simulink model "Wheel_NoneLinear_Verif"  (R2021b)
settings: Solver=VariableStepAuto  StartTime=0.0  StopTime=10  RelTol=1e-3
values from neighbouring files (symbols this model uses):
  Kt = 14e4    (= 140000)    [CarQuarterParam.m]
  M2 = 20    [CarQuarterParam.m]
settings Model: Creator=Reece Bell  LastModifiedBy=reece
settings SolverCC: AlgebraicLoopSolver=TrustRegion
settings DataIOCC: ReturnWorkspaceOutputs=off
settings DebuggingCC: SFMachineParentedDataDiag=warning  ArithmeticOperatorsInVariantConditions=warning
settings SFSimCC: CustomCodeUndefinedFunction=UseInterfaceOnly

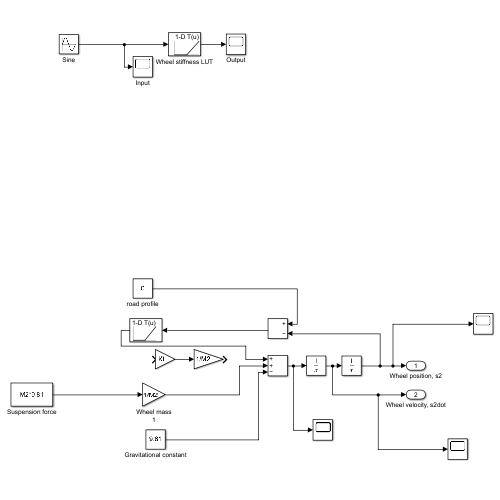
[thumbnail: Simulink's stored preview of the top-level diagram]
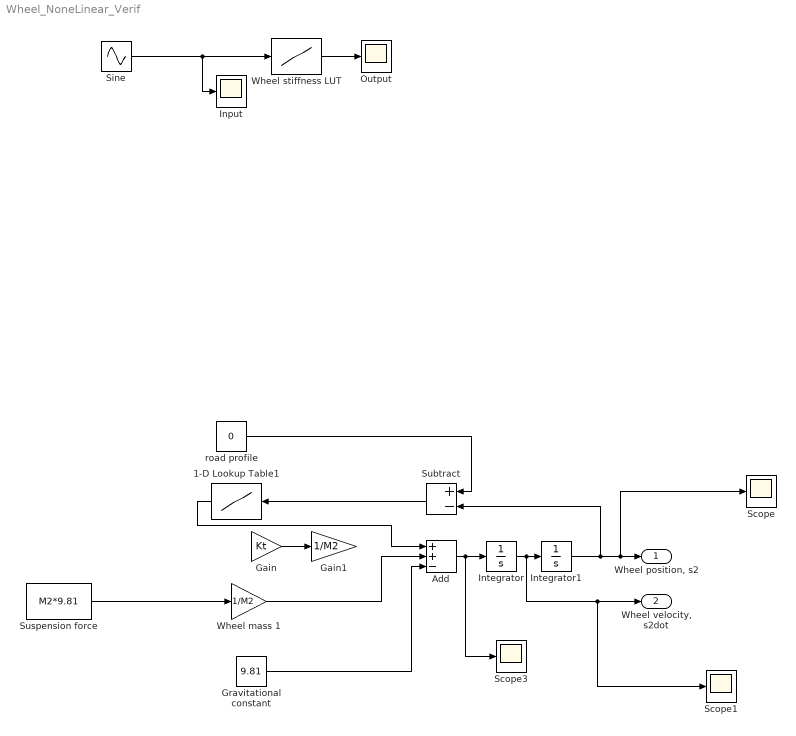
== system Wheel_NoneLinear_Verif ==
  1-D Lookup Table1 : Lookup_n-D  NumberOfTableDimensions=1  BreakpointsForDimension1=[-1,0,1]  Table=[0,0,Kt/M2]  InternalRulePriority=Speed  RndMeth=Simplest  InputSameDT=on
  Add : Sum  Inputs=++-
  Gain : Gain  Gain=Kt
  Gain1 : Gain  Gain=1/M2
  "Gravitational constant " : Constant  Value=9.81
  Input : Scope
  Integrator : Integrator
  Integrator1 : Integrator
  Output : Scope
  Scope : Scope
  Scope1 : Scope
  Scope3 : Scope
  Sine : Sin  SampleTime=0
  Subtract : Sum  Inputs=+-
  Suspension force : Constant  Value=M2*9.81
  Wheel mass 1 : Gain  Gain=1/M2
  Wheel stiffness LUT : Lookup_n-D  NumberOfTableDimensions=1  BreakpointsForDimension1=[-1,0,1]  Table=[0,0,Kt/M2]  InternalRulePriority=Speed  RndMeth=Simplest  InputSameDT=on
  road profile : Constant  Value=0
  "Wheel position, s2 " : Outport  VectorParamsAs1DForOutWhenUnconnected=off
  "Wheel velocity, s2dot " : Outport  Port=2  VectorParamsAs1DForOutWhenUnconnected=off
  wires:
  Suspension force/1 -> Wheel mass 1/1
  Integrator/1 -> Scope1/1, "Wheel velocity, s2dot "/1, Integrator1/1
  Wheel mass 1/1 -> Add/2
  "Gravitational constant "/1 -> Add/3
  Integrator1/1 -> Subtract/2, Scope/1, "Wheel position, s2 "/1
  Add/1 -> Scope3/1, Integrator/1
  Wheel stiffness LUT/1 -> Output/1
  Sine/1 -> Input/1, Wheel stiffness LUT/1
  Gain/1 -> Gain1/1
  Subtract/1 -> 1-D Lookup Table1/1
  1-D Lookup Table1/1 -> Add/1
  road profile/1 -> Subtract/1
